simulink model "kraefte_momente"  (R2025b)
settings: Solver=VariableStepAuto  StartTime=0.0  StopTime=10.0  RelTol=1e-3
undefined symbols (not defined in the file): Cd, g, m, MIX
settings Model: Creator=chris  LastModifiedBy=chris
settings ModelReferenceCC: ModelReferenceMinAlgLoopOccurrences=on

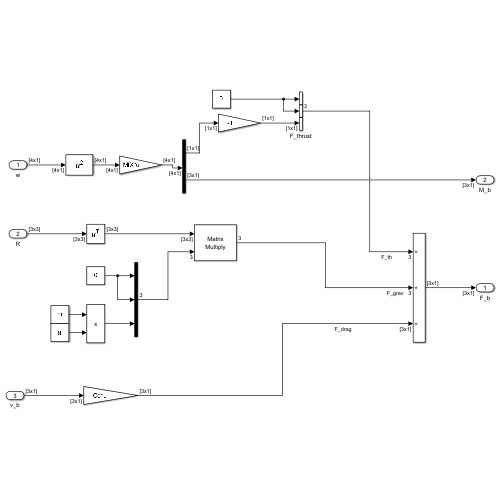
[thumbnail: Simulink's stored preview of the top-level diagram]
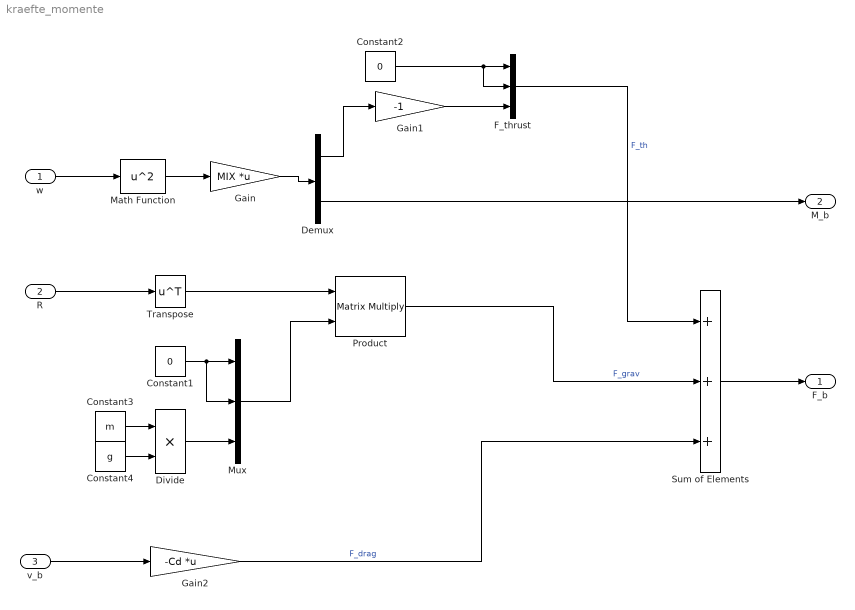
== system kraefte_momente ==
  w : Inport  PortDimensions=[4 1]
  R : Inport  Port=2  PortDimensions=[3 3]
  v_b : Inport  Port=3  PortDimensions=[3 1]
  Constant1 : Constant  Value=0
  Constant2 : Constant  Value=0
  Constant3 : Constant  Value=m
  Constant4 : Constant  Value=g
  Demux : Demux  Outputs=[1 3]
  Divide : Product  Inputs=**
  F_thrust : Concatenate  NumInputs=3
  Gain : Gain  Gain=MIX  Multiplication=Matrix(K*u)
  Gain1 : Gain  Gain=-1
  Gain2 : Gain  Gain=-Cd  Multiplication=Matrix(K*u)
  Math Function : Math  Operator=square
  Mux : Mux  Inputs=3
  Product : Product  Multiplication=Matrix(*)
  Sum of Elements : Sum  Inputs=+++
  Transpose : Math  Operator=transpose
  F_b : Outport  PortDimensions=[3 1]
  M_b : Outport  Port=2  PortDimensions=[3 1]
  wires:
  w/1 -> Math Function/1
  Math Function/1 -> Gain/1
  Gain/1 -> Demux/1
  Constant2/1 -> F_thrust/2, F_thrust/1
  Gain1/1 -> F_thrust/3
  Demux/1 -> Gain1/1
  Constant1/1 -> Mux/2, Mux/1
  Constant3/1 -> Divide/1
  Constant4/1 -> Divide/2
  R/1 -> Transpose/1
  Transpose/1 -> Product/1
  Mux/1 -> Product/2
  Sum of Elements/1 -> F_b/1
  v_b/1 -> Gain2/1
  Gain2/1 -> Sum of Elements/3  "F_drag"
  Product/1 -> Sum of Elements/2  "F_grav"
  Demux/2 -> M_b/1
  F_thrust/1 -> Sum of Elements/1  "F_th"
  Divide/1 -> Mux/3
